simulink library "MBDS_Modules"  (R2018b)
settings: Solver=ode45  StartTime=0.0  StopTime=10.0  RelTol=1e-3
libraries: simulink x1
Description:
  | MBDS project library for Module models
settings Model: Creator=uid60719  LastModifiedBy=uie79669
settings DataIOCC: LimitDataPoints=on  SaveFormat=Array  SignalLoggingSaveFormat=ModelDataLogs
settings OptimizationCC: BlockReduction=off  BooleanDataType=off  ExpressionDepthLimit=2147483647  LifeSpan=inf
settings DebuggingCC: SaveWithParameterizedLinksMsg=none  UnderspecifiedInitializationDetection=Classic  MergeDetectMultiDrivingBlocksExec=none  SignalResolutionControl=TryResolveAllWithWarning  MultiTaskCondExecSysMsg=none  FcnCallInpInsideContextMsg=warning  AllowSymbolicDim=off  StateNameClashWarn=warning  SFUnexpectedBacktrackingDiag=warning  SFNoUnconditionalDefaultTransitionDiag=warning  SFExecutionAtInitializationDiag=none
settings HardwareCC: ProdBitPerPointer=32  ProdBitPerSizeT=32  ProdBitPerPtrDiffT=32  ProdLargestAtomicFloat=None  ProdIntDivRoundTo=Undefined  ProdEndianess=Unspecified  ProdWordSize=32  ProdHWDeviceType=32-bit Generic  TargetUnknown=on
settings ModelReferenceCC: PropagateSignalLabelsOutOfModel=off
settings SFSimCC: SimUseLocalCustomCode=off
settings RTWCC: RTWUseLocalCustomCode=off
settings CodeAppCC: StateflowObjectComments=on
settings GRTTargetCC: TargetLangStandard=C89/C90 (ANSI)  GeneratePreprocessorConditionals=Disable all  CombineOutputUpdateFcns=off  GRTInterface=on
settings ConfigComp: CovMetricSettings=dw  CovHtmlReporting=on  CovSaveCumulativeToWorkspaceVar=on  CovSaveSingleToWorkspaceVar=on  CovExternalEMLEnable=off  CovSFcnEnable=off

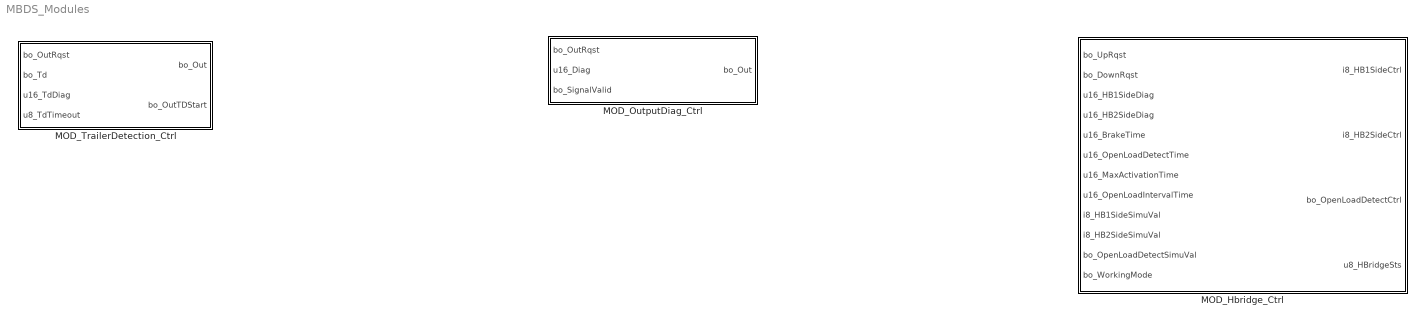
== system MBDS_Modules ==
  MOD_Hbridge_Ctrl : Subsystem  Description=Hbridge  mask(MOD_Hbridge_Ctrl){MBDS_ElementType=Module, MBDS_WorkStatus=In Work, MBDS_LastModified=2022-12-19-10:31:01}
      mask prompts: MBDS_ElementType "MBDS element type:"; MBDS_WorkStatus "Work status:"; MBDS_LastModified "Last modified:"
      mask help: Hbridge
      mask Help: eval(['open([workdir(''help_dir:''),''\MBDS_ProjectLibrary.html''])'])
      mask Display: disp('V 1.64')
  MOD_OutputDiag_Ctrl : Subsystem  Description=Controls output based on diagnostic signal  mask(MOD_OutputDiag_Ctrl){MBDS_ElementType=Module, MBDS_WorkStatus=In Work, MBDS_LastModified=2022-12-19-10:31:01}
      mask prompts: MBDS_ElementType "MBDS element type:"; MBDS_WorkStatus "Work status:"; MBDS_LastModified "Last modified:"
      mask help: Controls output based on diagnostic signal
      mask Help: eval(['open([workdir(''help_dir:''),''\MBDS_ProjectLibrary.html''])'])
      mask Display: disp('V 1.14')
  MOD_TrailerDetection_Ctrl : Subsystem  Description=Control outputs with Trailer detection hardware.  mask(MOD_TrailerDetection_Ctrl){MBDS_ElementType=Module, MBDS_WorkStatus=In Work, MBDS_LastModified=2022-12-19-10:31:00}
      mask prompts: MBDS_ElementType "MBDS element type:"; MBDS_WorkStatus "Work status:"; MBDS_LastModified "Last modified:"
      mask help: Control outputs with Trailer detection hardware.
      mask Help: eval(['open([workdir(''help_dir:''),''\MBDS_ProjectLibrary.html''])'])
      mask Display: disp('V 1.30')

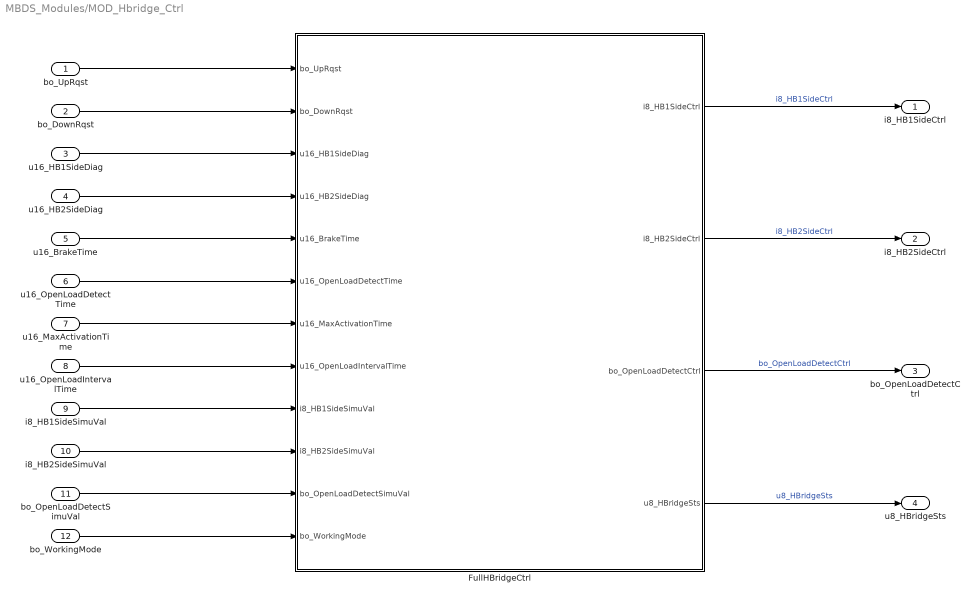
== system MBDS_Modules/MOD_Hbridge_Ctrl ==
  bo_UpRqst : Inport  OutDataTypeStr=boolean
  bo_DownRqst : Inport  Port=2  OutDataTypeStr=boolean
  u16_HB1SideDiag : Inport  Port=3  OutDataTypeStr=uint16
  u16_HB2SideDiag : Inport  Port=4  OutDataTypeStr=uint16
  u16_BrakeTime : Inport  Port=5  OutDataTypeStr=uint16
  u16_OpenLoadDetectTime : Inport  Port=6  OutDataTypeStr=uint16
  u16_MaxActivationTime : Inport  Port=7  OutDataTypeStr=uint16
  u16_OpenLoadIntervalTime : Inport  Port=8  OutDataTypeStr=uint16
  i8_HB1SideSimuVal : Inport  Port=9  OutDataTypeStr=int8
  i8_HB2SideSimuVal : Inport  Port=10  OutDataTypeStr=int8
  bo_OpenLoadDetectSimuVal : Inport  Port=11  OutDataTypeStr=boolean
  bo_WorkingMode : Inport  Port=12  OutDataTypeStr=boolean
  FullHBridgeCtrl : Stateflow chart  TreatAsAtomicUnit=on
      settings: CopyFcn=|
      | if(exist('MBDS_BlockCallback', 'file'))
      |    MBDS_BlockCallback('Copy', gcb);
      | end
  i8_HB1SideCtrl : Outport  OutDataTypeStr=int8
  i8_HB2SideCtrl : Outport  Port=2  OutDataTypeStr=int8
  bo_OpenLoadDetectCtrl : Outport  Port=3  OutDataTypeStr=boolean
  u8_HBridgeSts : Outport  Port=4  OutDataTypeStr=uint8
  wires:
  bo_WorkingMode/1 -> FullHBridgeCtrl/12(bo_WorkingMode)
  bo_OpenLoadDetectSimuVal/1 -> FullHBridgeCtrl/11(bo_OpenLoadDetectSimuVal)
  i8_HB2SideSimuVal/1 -> FullHBridgeCtrl/10(i8_HB2SideSimuVal)
  i8_HB1SideSimuVal/1 -> FullHBridgeCtrl/9(i8_HB1SideSimuVal)
  u16_OpenLoadIntervalTime/1 -> FullHBridgeCtrl/8(u16_OpenLoadIntervalTime)
  u16_MaxActivationTime/1 -> FullHBridgeCtrl/7(u16_MaxActivationTime)
  FullHBridgeCtrl/4(u8_HBridgeSts) -> u8_HBridgeSts/1  "u8_HBridgeSts"
  FullHBridgeCtrl/3(bo_OpenLoadDetectCtrl) -> bo_OpenLoadDetectCtrl/1  "bo_OpenLoadDetectCtrl"
  FullHBridgeCtrl/2(i8_HB2SideCtrl) -> i8_HB2SideCtrl/1  "i8_HB2SideCtrl"
  FullHBridgeCtrl/1(i8_HB1SideCtrl) -> i8_HB1SideCtrl/1  "i8_HB1SideCtrl"
  u16_OpenLoadDetectTime/1 -> FullHBridgeCtrl/6(u16_OpenLoadDetectTime)
  u16_BrakeTime/1 -> FullHBridgeCtrl/5(u16_BrakeTime)
  u16_HB2SideDiag/1 -> FullHBridgeCtrl/4(u16_HB2SideDiag)
  u16_HB1SideDiag/1 -> FullHBridgeCtrl/3(u16_HB1SideDiag)
  bo_DownRqst/1 -> FullHBridgeCtrl/2(bo_DownRqst)
  bo_UpRqst/1 -> FullHBridgeCtrl/1(bo_UpRqst)

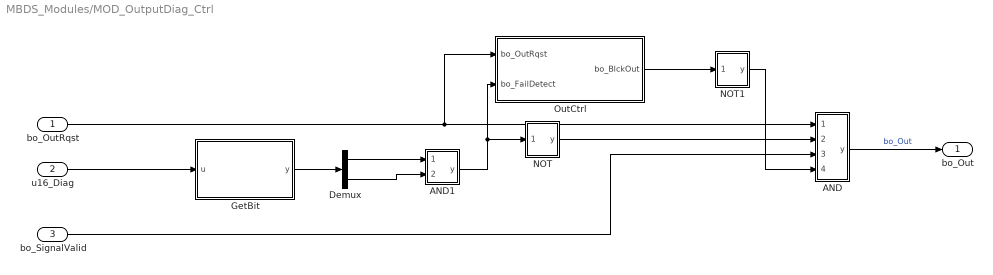
== system MBDS_Modules/MOD_OutputDiag_Ctrl ==
  bo_OutRqst : Inport  OutDataTypeStr=boolean
  u16_Diag : Inport  Port=2  OutDataTypeStr=uint16
  bo_SignalValid : Inport  Port=3  OutDataTypeStr=boolean
  AND : Subsystem  InitFcn=|  mask(AND){MBDS_LibraryBlock=on, BitwiseMode=off, Inputs=4, UseBitMask=off, BitMask='A7', OutDataTypeStr=Inherit: Inherit via back propagation, MBDS_BlockVersion=08.20.02}
      | if(exist('MBDS_BlockCallback', 'file'))
      |    MBDS_BlockCallback('Update', gcb);
      | end
      mask prompts: MBDS_LibraryBlock "MBDS library block"; BitwiseMode "Use 'bitwise' mode"; Inputs "Number of input ports:"; UseBitMask "Use bit mask"; BitMask "Bit mask:"; OutDataTypeStr "Output data type:"; MBDS_BlockVersion "Version:"
      mask help: Logical or bitwise AND operator. For multiple inputs, operators are applied across the inputs. For a single input, operators are applied across the input vector. In bitwise mode a bit mask can be applied onto single input signals.
      mask init:
      | if(exist('MBDS_BlockCallback', 'file'))
      |    MBDS_BlockCallback('Init', gcb);
      | else
      |    % Disable all mask parameters
      |    MaskEnables = get_param(gcb, 'MaskEnables');
      |    for k = [1:length(MaskEnables)]
      |       MaskEnables{k} = 'off';
      |    end
      |    if(~isequal(MaskEnables, get_param(gcb, 'MaskEnables')))
      |       set_param(gcb, 'MaskEnables', MaskEnables);
      |    end
      | end
      mask Help: eval(['open([workdir(''library_dir:''),''\Blockset\help\'',get_param(gcb,''MaskType''),''.html''])'])
      mask Callback BitwiseMode:
      | if(exist('MBDS_BlockCallback', 'file'))
      |    MBDS_BlockCallback('BitwiseMode', gcb);
      | end
      mask Callback Inputs:
      | if(exist('MBDS_BlockCallback', 'file'))
      |    MBDS_BlockCallback('Inputs', gcb);
      | end
      mask Callback UseBitMask:
      | if(exist('MBDS_BlockCallback', 'file'))
      |    MBDS_BlockCallback('UseBitMask', gcb);
      | end
      mask Callback BitMask:
      | if(exist('MBDS_BlockCallback', 'file'))
      |    MBDS_BlockCallback('BitMask', gcb);
      | end
      mask TypeOptions OutDataTypeStr: Inherit: Inherit via back propagation | int8 | uint8 | int16 | uint16 | int32 | uint32 | boolean
      mask Callback OutDataTypeStr:
      | % Adopt Value
      | if(exist('MBDS_BlockCallback', 'file'))
      |    MBDS_BlockCallback('OutDataTypeStr', gcb);
      | end
      mask DialogControl ParameterTabVar0 Prompt: Main
      mask DialogControl ParameterTabVar01 Prompt: Signal Attributes
      mask DialogControl ParameterTabVar012 Prompt: Version
      mask Display:
      | % Show icon or block text
      | if(UseBitMask)
      |    if(isnumeric(BitMask))
      |       BitMaskString = ['0x',dec2hex(floor(BitMask))];
      |    elseif(ischar(BitMask))
      |       BitMaskString = ['0x',upper(BitMask)];
      |    else
      |       BitMaskString = '???';
      |    end
      |    disp(sprintf(['AND\n', BitMaskString]))
      | else
      |    disp('AND')
      | end
  AND1 : Subsystem  InitFcn=|  mask(AND){MBDS_LibraryBlock=on, BitwiseMode=off, Inputs=2, UseBitMask=off, BitMask='A7', OutDataTypeStr=Inherit: Inherit via back propagation, MBDS_BlockVersion=08.20.02}
      | if(exist('MBDS_BlockCallback', 'file'))
      |    MBDS_BlockCallback('Update', gcb);
      | end
      mask prompts: MBDS_LibraryBlock "MBDS library block"; BitwiseMode "Use 'bitwise' mode"; Inputs "Number of input ports:"; UseBitMask "Use bit mask"; BitMask "Bit mask:"; OutDataTypeStr "Output data type:"; MBDS_BlockVersion "Version:"
      mask help: Logical or bitwise AND operator. For multiple inputs, operators are applied across the inputs. For a single input, operators are applied across the input vector. In bitwise mode a bit mask can be applied onto single input signals.
      mask init: same as MBDS_Modules/MOD_OutputDiag_Ctrl/AND
      mask Help: eval(['open([workdir(''library_dir:''),''\Blockset\help\'',get_param(gcb,''MaskType''),''.html''])'])
      mask Callback BitwiseMode:
      | if(exist('MBDS_BlockCallback', 'file'))
      |    MBDS_BlockCallback('BitwiseMode', gcb);
      | end
      mask Callback Inputs:
      | if(exist('MBDS_BlockCallback', 'file'))
      |    MBDS_BlockCallback('Inputs', gcb);
      | end
      mask Callback UseBitMask:
      | if(exist('MBDS_BlockCallback', 'file'))
      |    MBDS_BlockCallback('UseBitMask', gcb);
      | end
      mask Callback BitMask:
      | if(exist('MBDS_BlockCallback', 'file'))
      |    MBDS_BlockCallback('BitMask', gcb);
      | end
      mask TypeOptions OutDataTypeStr: Inherit: Inherit via back propagation | int8 | uint8 | int16 | uint16 | int32 | uint32 | boolean
      mask Callback OutDataTypeStr:
      | % Adopt Value
      | if(exist('MBDS_BlockCallback', 'file'))
      |    MBDS_BlockCallback('OutDataTypeStr', gcb);
      | end
      mask DialogControl ParameterTabVar0 Prompt: Main
      mask DialogControl ParameterTabVar01 Prompt: Signal Attributes
      mask DialogControl ParameterTabVar012 Prompt: Version
      mask Display:
      | % Show icon or block text
      | if(UseBitMask)
      |    if(isnumeric(BitMask))
      |       BitMaskString = ['0x',dec2hex(floor(BitMask))];
      |    elseif(ischar(BitMask))
      |       BitMaskString = ['0x',upper(BitMask)];
      |    else
      |       BitMaskString = '???';
      |    end
      |    disp(sprintf(['AND\n', BitMaskString]))
      | else
      |    disp('AND')
      | end
  Demux : Demux  InitFcn=|  Outputs=2
      | try
      |    MBDS_BlockCallback('Update', gcb);
      | end
  GetBit : Subsystem  InitFcn=|  mask(GetBit){MBDS_LibraryBlock=on, ZeroIndexing=on, SEL_Enabled=off, SEL=[7 12], MBDS_BlockVersion=08.20.02}
      | if(exist('MBDS_BlockCallback', 'file'))
      |    MBDS_BlockCallback('Update', gcb);
      | end
      mask prompts: MBDS_LibraryBlock "MBDS library block"; ZeroIndexing "Use zero-based indexing"; SEL_Enabled "Show SEL port"; SEL "Bit selection:"; MBDS_BlockVersion "Block version:"
      mask help: Get the value of the specified bit from the input signal.
      mask init: same as MBDS_Modules/MOD_OutputDiag_Ctrl/AND
      settings: AttributesFormatString=Zero-based indexing: %<ZeroIndexing>
      mask Help: eval(['open([workdir(''library_dir:''),''\Blockset\help\'',get_param(gcb,''MaskType''),''.html''])'])
      mask Callback ZeroIndexing:
      | % Adopt Value
      | if(exist('MBDS_BlockCallback', 'file'))
      |    MBDS_BlockCallback('ZeroIndexing', gcb);
      | end
      mask Callback SEL_Enabled:
      | % Update mask parameter dialog
      | if(exist('MBDS_BlockCallback', 'file'))
      |    MBDS_BlockCallback('SEL_Enabled', gcb);
      | end
      mask Callback SEL:
      | % Adopt Value
      | if(exist('MBDS_BlockCallback', 'file'))
      |    MBDS_BlockCallback('SEL', gcb);
      | end
      mask DialogControl ParameterTabVar0 Prompt: Main
      mask DialogControl ParameterTabVar01 Prompt: Version
      mask Display:
      | % Show block text
      | disp(sprintf('Get Bit'));
      | 
      | % Display port labels
      | port_label('input', 1, 'u');
      | port_label('output', 1, 'y');
  NOT : Subsystem  InitFcn=|  mask(NOT){MBDS_LibraryBlock=on, BitwiseMode=off, Inputs=1, UseBitMask=off, BitMask='A1', OutDataTypeStr=Inherit: Inherit via back propagation, MBDS_BlockVersion=08.20.02}
      | if(exist('MBDS_BlockCallback', 'file'))
      |    MBDS_BlockCallback('Update', gcb);
      | end
      mask prompts: MBDS_LibraryBlock "MBDS library block"; BitwiseMode "Use 'bitwise' mode"; Inputs "Number of input ports:"; UseBitMask "Use bit mask"; BitMask "Bit mask:"; OutDataTypeStr "Output data type:"; MBDS_BlockVersion "Version:"
      mask help: Logical or bitwise NOT operator. The input value is inverted. In bitwise mode all bits of the input signal are inverted.
      mask init: same as MBDS_Modules/MOD_OutputDiag_Ctrl/AND
      mask Help: eval(['open([workdir(''library_dir:''),''\Blockset\help\'',get_param(gcb,''MaskType''),''.html''])'])
      mask Callback BitwiseMode:
      | if(exist('MBDS_BlockCallback', 'file'))
      |    MBDS_BlockCallback('BitwiseMode', gcb);
      | end
      mask TypeOptions OutDataTypeStr: Inherit: Inherit via back propagation | int8 | uint8 | int16 | uint16 | int32 | uint32 | boolean
      mask Callback OutDataTypeStr:
      | % Adopt Value
      | if(exist('MBDS_BlockCallback', 'file'))
      |    MBDS_BlockCallback('OutDataTypeStr', gcb);
      | end
      mask DialogControl ParameterTabVar0 Prompt: Main
      mask DialogControl ParameterTabVar01 Prompt: Signal Attributes
      mask DialogControl ParameterTabVar012 Prompt: Version
      mask Display:
      | % Show icon or block text
      | disp('NOT')
  NOT1 : Subsystem  InitFcn=|  mask(NOT){MBDS_LibraryBlock=on, BitwiseMode=off, Inputs=1, UseBitMask=off, BitMask='A1', OutDataTypeStr=Inherit: Inherit via back propagation, MBDS_BlockVersion=08.20.02}
      | if(exist('MBDS_BlockCallback', 'file'))
      |    MBDS_BlockCallback('Update', gcb);
      | end
      mask prompts: MBDS_LibraryBlock "MBDS library block"; BitwiseMode "Use 'bitwise' mode"; Inputs "Number of input ports:"; UseBitMask "Use bit mask"; BitMask "Bit mask:"; OutDataTypeStr "Output data type:"; MBDS_BlockVersion "Version:"
      mask help: Logical or bitwise NOT operator. The input value is inverted. In bitwise mode all bits of the input signal are inverted.
      mask init: same as MBDS_Modules/MOD_OutputDiag_Ctrl/AND
      mask Help: eval(['open([workdir(''library_dir:''),''\Blockset\help\'',get_param(gcb,''MaskType''),''.html''])'])
      mask Callback BitwiseMode:
      | if(exist('MBDS_BlockCallback', 'file'))
      |    MBDS_BlockCallback('BitwiseMode', gcb);
      | end
      mask TypeOptions OutDataTypeStr: Inherit: Inherit via back propagation | int8 | uint8 | int16 | uint16 | int32 | uint32 | boolean
      mask Callback OutDataTypeStr:
      | % Adopt Value
      | if(exist('MBDS_BlockCallback', 'file'))
      |    MBDS_BlockCallback('OutDataTypeStr', gcb);
      | end
      mask DialogControl ParameterTabVar0 Prompt: Main
      mask DialogControl ParameterTabVar01 Prompt: Signal Attributes
      mask DialogControl ParameterTabVar012 Prompt: Version
      mask Display:
      | % Show icon or block text
      | disp('NOT')
  OutCtrl : Stateflow chart  TreatAsAtomicUnit=on
      settings: CopyFcn=|
      | if(exist('MBDS_BlockCallback', 'file'))
      |    MBDS_BlockCallback('Copy', gcb);
      | end
  bo_Out : Outport  OutDataTypeStr=boolean
  wires:
  NOT1/1(y) -> AND/4(u4)
  OutCtrl/1(bo_BlckOut) -> NOT1/1(u1)
  NOT/1(y) -> AND/2(u2)
  AND1/1(y) -> NOT/1(u1), OutCtrl/2(bo_FailDetect)
  bo_SignalValid/1 -> AND/3(u3)
  Demux/2 -> AND1/2(u2)
  Demux/1 -> AND1/1(u1)
  GetBit/1(y) -> Demux/1
  AND/1(y) -> bo_Out/1  "bo_Out"
  u16_Diag/1 -> GetBit/1(u)
  bo_OutRqst/1 -> AND/1(u1), OutCtrl/1(bo_OutRqst)

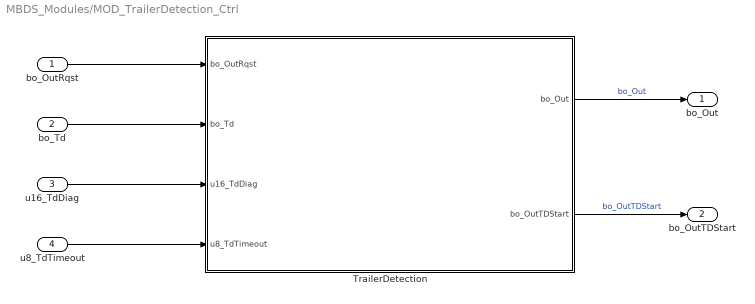
== system MBDS_Modules/MOD_TrailerDetection_Ctrl ==
  bo_OutRqst : Inport  OutDataTypeStr=boolean
  bo_Td : Inport  Port=2  OutDataTypeStr=boolean
  u16_TdDiag : Inport  Port=3  OutDataTypeStr=uint16
  u8_TdTimeout : Inport  Port=4  OutDataTypeStr=uint8
  TrailerDetection : Stateflow chart  TreatAsAtomicUnit=on
      settings: CopyFcn=|
      | if(exist('MBDS_BlockCallback', 'file'))
      |    MBDS_BlockCallback('Copy', gcb);
      | end
  bo_Out : Outport  OutDataTypeStr=boolean
  bo_OutTDStart : Outport  Port=2  OutDataTypeStr=boolean
  wires:
  u8_TdTimeout/1 -> TrailerDetection/4(u8_TdTimeout)
  TrailerDetection/2(bo_OutTDStart) -> bo_OutTDStart/1  "bo_OutTDStart"
  TrailerDetection/1(bo_Out) -> bo_Out/1  "bo_Out"
  u16_TdDiag/1 -> TrailerDetection/3(u16_TdDiag)
  bo_Td/1 -> TrailerDetection/2(bo_Td)
  bo_OutRqst/1 -> TrailerDetection/1(bo_OutRqst)

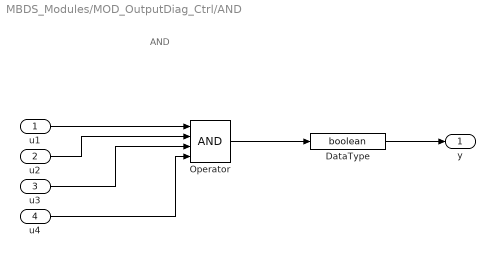
== system MBDS_Modules/MOD_OutputDiag_Ctrl/AND ==
  note: AND
  u1 : Inport  OutDataTypeStr=boolean
  u2 : Inport  Port=2  OutDataTypeStr=boolean
  u3 : Inport  Port=3  OutDataTypeStr=boolean
  u4 : Inport  Port=4  OutDataTypeStr=boolean
  DataType : DataTypeConversion  OutDataTypeStr=boolean
  Operator : Logic  Inputs=4  AllPortsSameDT=off  OutDataTypeStr=boolean
  y : Outport
  wires:
  u4/1 -> Operator/4
  u3/1 -> Operator/3
  DataType/1 -> y/1
  u2/1 -> Operator/2
  u1/1 -> Operator/1
  Operator/1 -> DataType/1

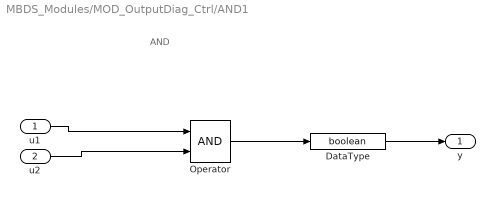
== system MBDS_Modules/MOD_OutputDiag_Ctrl/AND1 ==
  note: AND
  u1 : Inport  OutDataTypeStr=boolean
  u2 : Inport  Port=2  OutDataTypeStr=boolean
  DataType : DataTypeConversion  OutDataTypeStr=boolean
  Operator : Logic  AllPortsSameDT=off  OutDataTypeStr=boolean
  y : Outport
  wires:
  DataType/1 -> y/1
  u2/1 -> Operator/2
  u1/1 -> Operator/1
  Operator/1 -> DataType/1

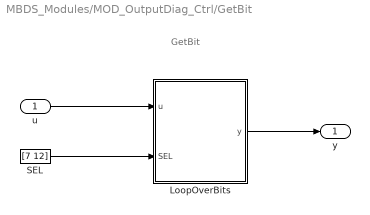
== system MBDS_Modules/MOD_OutputDiag_Ctrl/GetBit ==
  note: GetBit
  u : Inport
  LoopOverBits : Subsystem
  SEL : Constant  Value=[7 12]  OutDataTypeStr=uint8
  y : Outport
  wires:
  LoopOverBits/1(y) -> y/1
  SEL/1 -> LoopOverBits/2(SEL)
  u/1 -> LoopOverBits/1(u)

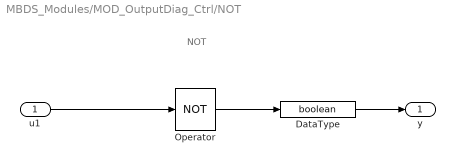
== system MBDS_Modules/MOD_OutputDiag_Ctrl/NOT ==
  note: NOT
  u1 : Inport  OutDataTypeStr=boolean
  DataType : DataTypeConversion  OutDataTypeStr=boolean
  Operator : Logic  Operator=NOT  Inputs=1  AllPortsSameDT=off  OutDataTypeStr=boolean
  y : Outport
  wires:
  DataType/1 -> y/1
  u1/1 -> Operator/1
  Operator/1 -> DataType/1

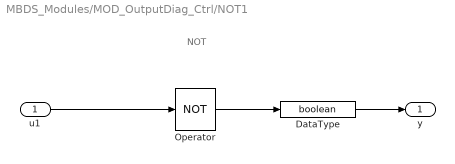
== system MBDS_Modules/MOD_OutputDiag_Ctrl/NOT1 ==
  note: NOT
  u1 : Inport  OutDataTypeStr=boolean
  DataType : DataTypeConversion  OutDataTypeStr=boolean
  Operator : Logic  Operator=NOT  Inputs=1  AllPortsSameDT=off  OutDataTypeStr=boolean
  y : Outport
  wires:
  DataType/1 -> y/1
  u1/1 -> Operator/1
  Operator/1 -> DataType/1

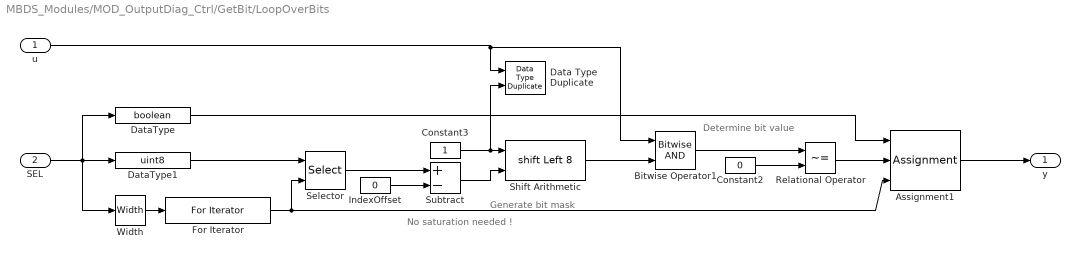
== system MBDS_Modules/MOD_OutputDiag_Ctrl/GetBit/LoopOverBits ==
  note: No saturation
      | needed !
  note: Determine bit value
  note: Generate bit mask
  u : Inport
  SEL : Inport  Port=2
  Assignment1 : Assignment  IndexMode=Zero-based  IndexOptions=Index vector (port)  Indices=1  OutputSizes=[1 1]
  Bitwise Operator1 : simulink/Logic and Bit Operations/Bitwise Operator  logicop=AND  UseBitMask=off  NumInputPorts=2  BitMask=bin2dec('11011001')  BitMaskRealWorld=Stored Integer
  Constant2 : Constant  Value=0  OutDataTypeStr=Inherit: Inherit via back propagation
  Constant3 : Constant  OutDataTypeStr=Inherit: Inherit via back propagation
  Data Type Duplicate : DataTypeDuplicate  InitFcn=|
      | try
      |    MBDS_BlockCallback('Update', gcb);
      | end
  DataType : DataTypeConversion  OutDataTypeStr=boolean
  DataType1 : DataTypeConversion  OutDataTypeStr=uint8
  For Iterator : ForIterator  IterationSource=external  IndexMode=Zero-based  IterationVariableDataType=int8
  IndexOffset : Constant  Value=0  OutDataTypeStr=Inherit: Inherit via back propagation
  Relational Operator : RelationalOperator  Operator=~=  OutDataTypeStr=boolean  RndMeth=Nearest
  Selector : Selector  IndexMode=Zero-based  IndexOptions=Index vector (port)  Indices=[1 3]  OutputSizes=1
  Shift Arithmetic : ArithShift  BitShiftNumberSource=Input port  BitShiftNumber=8  BitShiftDirection=Left
      settings: InputPortMap=u0,p1
  Subtract : Sum  Inputs=+-  OutDataTypeStr=Inherit: Inherit via back propagation  InputSameDT=on
  Width : Width  DataType=uint8
  y : Outport
  wires:
  u/1 -> Data Type Duplicate/1, Bitwise Operator1/1
  DataType1/1 -> Selector/1
  SEL/1 -> Width/1, DataType/1, DataType1/1
  DataType/1 -> Assignment1/1
  Assignment1/1 -> y/1
  Relational Operator/1 -> Assignment1/2
  Constant2/1 -> Relational Operator/2
  Bitwise Operator1/1 -> Relational Operator/1
  Shift Arithmetic/1 -> Bitwise Operator1/2
  Constant3/1 -> Data Type Duplicate/2, Shift Arithmetic/1
  Width/1 -> For Iterator/1
  For Iterator/1 -> Assignment1/3, Selector/2
  Selector/1 -> Subtract/1
  Subtract/1 -> Shift Arithmetic/2
  IndexOffset/1 -> Subtract/2

== stateflow chart MBDS_Modules/MOD_OutputDiag_Ctrl/OutCtrl ==
  state OutOn
  state Wait
    en:
    bo_BlckOut = false;
  state BlockOutput
    en:
    bo_BlckOut = true;
  Wait -> OutOn : [bo_OutRqst == true]
  OutOn -> BlockOutput [order 1] : [bo_FailDetect == true]
  (default) -> Wait
  OutOn -> Wait [order 2] : [bo_OutRqst == false]
  BlockOutput -> Wait : [bo_OutRqst == false]
  data: bo_OutRqst input boolean; bo_FailDetect input boolean; bo_BlckOut output boolean

== stateflow chart MBDS_Modules/MOD_Hbridge_Ctrl/FullHBridgeCtrl ==
  state H_SimulationMode
    en:
    u8_HBridgeSts= u8_HSimu;
    i8_HB1SideCtrl = i8_HBOFF;
    i8_HB2SideCtrl = i8_HBOFF;
    bo_OpenLoadDetectCtrl=false;
    du:
    i8_HB1SideCtrl = i8_HB1SideSimuVal;
    i8_HB2SideCtrl = i8_HB2SideSimuVal;
    bo_OpenLoadDetectCtrl=bo_OpenLoadDetectSimuVal;
  state H_StandAlone
    state H_ForceBrake
      en:
      u16_Timer=uint16(1);
      u8_HBridgeSts= u8_HForceBrake;
      i8_HB1SideCtrl = i8_HBLS;
      i8_HB2SideCtrl = i8_HBLS;
      bo_OpenLoadDetectCtrl=false;
      du:
      u16_Timer++;
    state H_OFF
      en:
      u16_Timer=uint16(1);
      u8_HBridgeSts= u8_HOFF;
      i8_HB1SideCtrl = i8_HBOFF;
      i8_HB2SideCtrl = i8_HBOFF;
      bo_OpenLoadDetectCtrl=false;
      du:
      u16_Timer++;
    state H_Failure
      en:
      u8_HBridgeSts= u8_HFail;
      i8_HB1SideCtrl = i8_HBOFF;
      i8_HB2SideCtrl = i8_HBOFF;
      bo_OpenLoadDetectCtrl=false;
    state H_OLD
      en:
      u16_Timer=uint16(1);
      u8_HBridgeSts= u8_HOLD;
      i8_HB1SideCtrl = i8_HBLS;
      i8_HB2SideCtrl = i8_HBOFF;
      bo_OpenLoadDetectCtrl=true;
      du:
      u16_Timer++;
    state H_WaitForNoRqst
      en:
      u8_HBridgeSts= u8_HWait;
      i8_HB1SideCtrl = i8_HBOFF;
      i8_HB2SideCtrl = i8_HBOFF;
      bo_OpenLoadDetectCtrl=false;
    state H_Down
      en:
      u16_Timer=uint16(1);
      u8_HBridgeSts= u8_HDown;
      i8_HB1SideCtrl = i8_HBOFF;
      i8_HB2SideCtrl = i8_HBOFF;
      bo_OpenLoadDetectCtrl=false;
      du:
      i8_HB1SideCtrl = i8_HBLS;
      i8_HB2SideCtrl = i8_HBHS;
      u16_Timer++;
    state H_Up
      en:
      u16_Timer=uint16(1);
      u8_HBridgeSts= u8_HUp;
      i8_HB1SideCtrl = i8_HBOFF;
      i8_HB2SideCtrl = i8_HBOFF;
      bo_OpenLoadDetectCtrl=false;
      du:
      i8_HB1SideCtrl = i8_HBHS;
      i8_HB2SideCtrl = i8_HBLS;
      u16_Timer++;
    state H_Brake
      en:
      u16_Timer=uint16(1);
      u8_HBridgeSts= u8_HBrake;
      i8_HB1SideCtrl = i8_HBLS;
      i8_HB2SideCtrl = i8_HBLS;
      bo_OpenLoadDetectCtrl=false;
      du:
      u16_Timer++;
    (default) -> H_ForceBrake
    H_Failure -> H_OFF : /* Request to turn H bridge OFF*/
        | [bo_UpRqst == false && bo_DownRqst == false]
    H_ForceBrake -> H_WaitForNoRqst : [u16_Timer >= u16_BrakeTime]
    H_OFF -> H_OLD : /* Request to turn H bridge ON or OLD intervaltime*/
        | [bo_UpRqst == true ||...
        | bo_DownRqst == true ||...
        | u16_Timer >= u16_OpenLoadIntervalTime]
    H_OLD -> H_Failure [order 1] : /* Open Load Detected */
        | [u16_Timer >= u16_OpenLoadDetectTime&&...
        | (u16_HB1SideDiag!=uint16(0x0000)||...
        | u16_HB2SideDiag!=uint16(0x0000))]
    H_WaitForNoRqst -> H_OFF : /* Wait till no Request to avoid start
        | moving actuators after POR*/
        | [bo_UpRqst == false &&...
        | bo_DownRqst == false]
    H_OLD -> H_OFF [order 2] : /* No Request to turn H bridge ON*/
        | [bo_UpRqst == false &&...
        | bo_DownRqst == false&&...
        | u16_Timer >= u16_OpenLoadDetectTime]
    H_OLD -> H_Up [order 3] : /* Up Rqst - OLD not Detected */
        | [bo_UpRqst == true&&...
        | bo_DownRqst == false&&...
        | u16_Timer >= u16_OpenLoadDetectTime]
    H_OLD -> H_Down [order 4] : /* Down Rqst - OLD not Detected */
        | [bo_UpRqst == false&&...
        | bo_DownRqst == true&&...
        | u16_Timer >= u16_OpenLoadDetectTime]
    H_Up -> H_Brake : /* Up Not Rqst or Timeout or error */
        | [bo_UpRqst == false ||...
        | u16_HB1SideDiag!=uint16(0x0000)||...
        | u16_HB2SideDiag!=uint16(0x0000)||...
        | u16_Timer >= u16_MaxActivationTime]
    H_Brake -> H_Up [order 2] : /* Up Request after Brake*/
        | [bo_UpRqst == true&&...
        | bo_DownRqst == false&&...
        | u16_Timer >= u16_BrakeTime]
    H_Brake -> H_Down [order 3] : /* Down Request after Brake */
        | [bo_UpRqst == false&&...
        | bo_DownRqst == true&&...
        | u16_Timer >= u16_BrakeTime]
    H_Down -> H_Brake : /* Down Not Rqst or Timeout  or error*/
        | [bo_DownRqst == false ||...
        | u16_HB1SideDiag!=uint16(0x0000)||...
        | u16_HB2SideDiag!=uint16(0x0000)||...
        | u16_Timer >= u16_MaxActivationTime]
    H_Brake -> H_OFF [order 4] : /* Request to turn H bridge OFF  after Brake*/
        | [bo_UpRqst == false &&...
        |  bo_DownRqst == false &&...
        | u16_Timer >= u16_BrakeTime]
    H_Brake -> H_Failure [order 1] : /* Failure Detected after Brake */
        | [u16_Timer >= u16_BrakeTime&&...
        | (u16_HB1SideDiag!=uint16(0x0000)||...
        | u16_HB2SideDiag!=uint16(0x0000))]
  state H_SimulationBrake
    en:
    u16_Timer=uint16(1);
    u8_HBridgeSts= u8_HBrakeSimulation;
    i8_HB1SideCtrl = i8_HBLS;
    i8_HB2SideCtrl = i8_HBLS;
    bo_OpenLoadDetectCtrl=false;
    du:
    u16_Timer++;
  (default) -> H_SimulationMode
  H_SimulationMode -> H_StandAlone : [bo_WorkingMode==true]
  H_SimulationBrake -> H_SimulationMode : [u16_Timer >= u16_BrakeTime]
  H_StandAlone -> H_SimulationBrake : [bo_WorkingMode==false]
  data: bo_UpRqst input boolean; bo_DownRqst input boolean; i8_HB1SideCtrl output int8 =0; i8_HB2SideCtrl output int8 =0; u16_Timer local uint16 =0; u16_HB1SideDiag input uint16; u16_HB2SideDiag input uint16; u16_BrakeTime input uint16; bo_OpenLoadDetectCtrl output boolean =false; u16_OpenLoadDetectTime input uint16; u8_HBridgeSts output uint8 =0; i8_HBHS local int8 =1; i8_HBLS local int8 =-1; i8_HBOFF local int8 =0; u8_HOFF local uint8 =0; u8_HBrake local uint8 =1; u8_HOLD local uint8 =2; u8_HUp local uint8 =3; u8_HDown local uint8 =4; u8_HFail local uint8 =5; u16_MaxActivationTime input uint16; u16_OpenLoadIntervalTime input uint16; u8_HWait local uint8 =6; i8_HB1SideSimuVal input int8; i8_HB2SideSimuVal input int8; bo_OpenLoadDetectSimuVal input boolean; bo_WorkingMode input boolean; u8_HSimu local uint8 =7; u8_HForceBrake local uint8 =8; u8_HBrakeSimulation local uint8 =9

== stateflow chart MBDS_Modules/MOD_TrailerDetection_Ctrl/TrailerDetection ==
  state OUT_OFF
    en:
    u8_Timer=0;
    bo_Out = false;
    bo_OutTDStart = false;
  state TD_Start
    en:
    bo_OutTDStart = true;
    u8_Timer=0;
    du:
    u8_Timer++;
  state OUT_ON
    en:
    bo_OutTDStart = false;
    bo_Out = true;
  (default) -> OUT_OFF
  OUT_OFF -> TD_Start : /* Out off and requested to turn ON */
      | [bo_OutRqst == true]
  TD_Start -> OUT_OFF [order 1] : /* Output request is OFF*/
      | [bo_OutRqst == false]
  TD_Start -> OUT_ON [order 2] : /* Timer elapsed */
      | [u8_Timer > u8_TdTimeout]
  OUT_ON -> OUT_OFF : /* Output request OFF */
      | [bo_OutRqst == false]
  data: bo_OutRqst input boolean; bo_Out output boolean =false; u8_Timer local uint8 =0; bo_Td input boolean; u16_TdDiag input uint16; bo_OutTDStart output boolean =false; u8_TdTimeout input uint8
